simulink model "CPR_Controller"  (R2024b)
settings: Solver=VariableStepAuto  StartTime=0.0  StopTime=3  MaxStep=0.00001  RelTol=1e-6
values from neighbouring files (symbols this model uses):
  k = 1    [nyqlog.m]
  R = R/spiralfactor    (= 6.66666666667e-06)    [nyqlog.m]
undefined symbols (not defined in the file or in its folder): alpha, b, c, denom_discrete, dspblkCoreblockFVToolHelper, gcbh, J, K_i, K_p, K_torque, m, num_discrete, plant_denom, plant_num, T, tau
libraries: dspstat3 x1, dspsigops x1
settings Model: Creator=jonat  LastModifiedBy=jonat

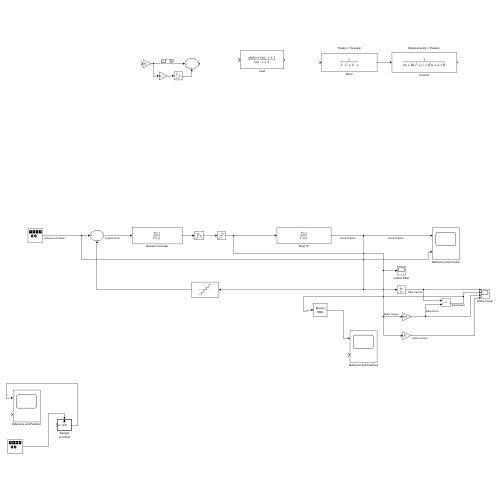
[thumbnail: Simulink's stored preview of the top-level diagram]
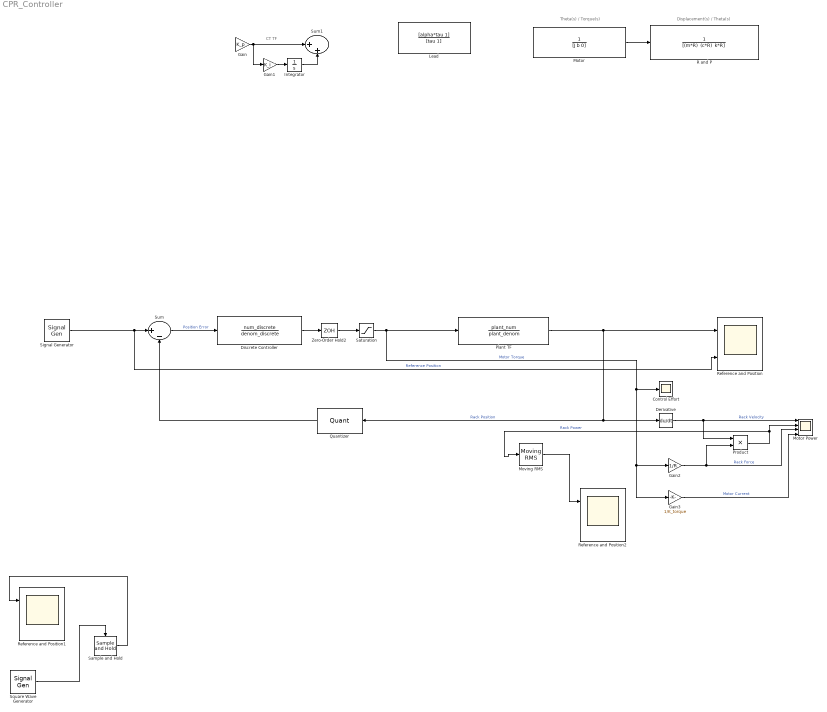
== system CPR_Controller ==
  note: CT TF
  note: Displacement(s) / Theta(s)
  note: Theta(s) / Torque(s)
  Control Effort : Scope
  Derivative : Derivative
  Discrete Controller : DiscreteTransferFcn  LoadFcn=dspblkCoreblockFVToolHelper(gcbh,'load');  Numerator=num_discrete  Denominator=denom_discrete
      settings: CopyFcn=dspblkCoreblockFVToolHelper(gcbh,'copy');  DeleteFcn=dspblkCoreblockFVToolHelper(gcbh,'close');  ModelCloseFcn=dspblkCoreblockFVToolHelper(gcbh,'close');  PreSaveFcn=dspblkCoreblockFVToolHelper(gcbh,'presave');  PostSaveFcn=dspblkCoreblockFVToolHelper(gcbh,'postsave');  CloseFcn=dspblkCoreblockFVToolHelper(gcbh,'close');
  Gain : Gain  Gain=K_p
  Gain1 : Gain  Gain=K_i
  Gain2 : Gain  Gain=1/R
  Gain3 : Gain  Gain=1/K_torque
  Integrator : Integrator  LimitOutput=on  UpperSaturationLimit=5  LowerSaturationLimit=-5
  Lead : TransferFcn  Numerator=[alpha*tau 1]  Denominator=[tau 1]
  Motor : TransferFcn  Denominator=[J b 0]
  Motor Power : Scope  NumInputPorts=4
  Moving RMS : dspstat3/Moving RMS  Method=Sliding window  ForgettingFactorPort=off  SpecifyWindowLength=on  WindowLength=4  OverlapLength=3  AllowArbitraryInputLength=off  ForgettingFactor=0.9  SimulateUsing=Interpreted execution
  Plant TF : TransferFcn  Numerator=plant_num  Denominator=plant_denom
  Product : Product
  Quantizer : Quantizer  QuantizationInterval=0.0005
  R and P : TransferFcn  Denominator="[(m*R)  (c*R)  k*R]"
  Reference and Position : Scope  NumInputPorts=2
  Reference and Position1 : Scope  NumInputPorts=2
  Reference and Position2 : Scope  NumInputPorts=2
  Sample and Hold : dspsigops/Sample and Hold  trig=Rising edge  initCond=0  latchinput=off
  Saturation : Saturate  UpperLimit=5  LowerLimit=-5
  Signal Generator : SignalGenerator  Amplitude=.05/2  Frequency=2
  Square Wave Generator : SignalGenerator  WaveForm=square  Frequency=1/T
  Sum : Sum  Inputs=|+-
  Sum1 : Sum  Inputs=|++
  Zero-Order Hold2 : ZeroOrderHold  SampleTime=T
  wires:
  Plant TF/1 -> Quantizer/1, Derivative/1, Reference and Position/1  "Rack Position"
  Motor/1 -> R and P/1
  Square Wave Generator/1 -> Sample and Hold/Trigger
  Sample and Hold/1 -> Reference and Position1/1
  Gain1/1 -> Integrator/1
  Gain/1 -> Gain1/1, Sum1/1
  Integrator/1 -> Sum1/2
  Saturation/1 -> Gain3/1, Gain2/1, Control Effort/1, Plant TF/1  "Motor Torque"
  Derivative/1 -> Product/1, Motor Power/1  "Rack Velocity"
  Gain2/1 -> Product/2, Motor Power/3  "Rack Force"
  Product/1 -> Moving RMS/1, Motor Power/2  "Rack Power"
  Quantizer/1 -> Sum/2
  Sum/1 -> Discrete Controller/1  "Position Error"
  Discrete Controller/1 -> Zero-Order Hold2/1
  Signal Generator/1 -> Reference and Position/2, Sum/1  "Reference Position"
  Zero-Order Hold2/1 -> Saturation/1
  Gain3/1 -> Motor Power/4  "Motor Current"
  Moving RMS/1 -> Reference and Position2/1
